simulink model "Hava_Araci_6DOF"  (R2022a)
settings: Solver=ode4  StartTime=0.0  StopTime=inf  FixedStep=1/1000  RelTol=1e-3
InitFcn:
  | addpath(genpath(cd))
  | run('Konfig_Yukle.m')
undefined symbols (not defined in the file or in its folder): aerodatabase, ataletsel, baslangic, e0_0, e1_0, e2_0, e3_0, itki, pm_0, servo, sevo, Vm_0, xme_0
libraries: simulink_extras x9, sharedtransform x3, matrix_library x2, vrlib x1, aerolibtransform2 x1, aerolibatmos2 x1, dspnetwork x1
settings Model: Creator=Fatabi  LastModifiedBy=Fatabi

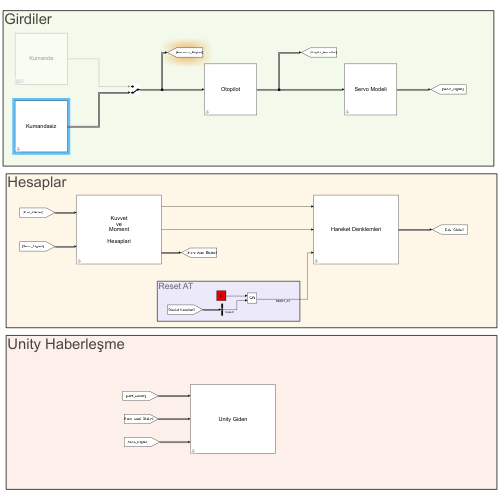
[thumbnail: Simulink's stored preview of the top-level diagram]
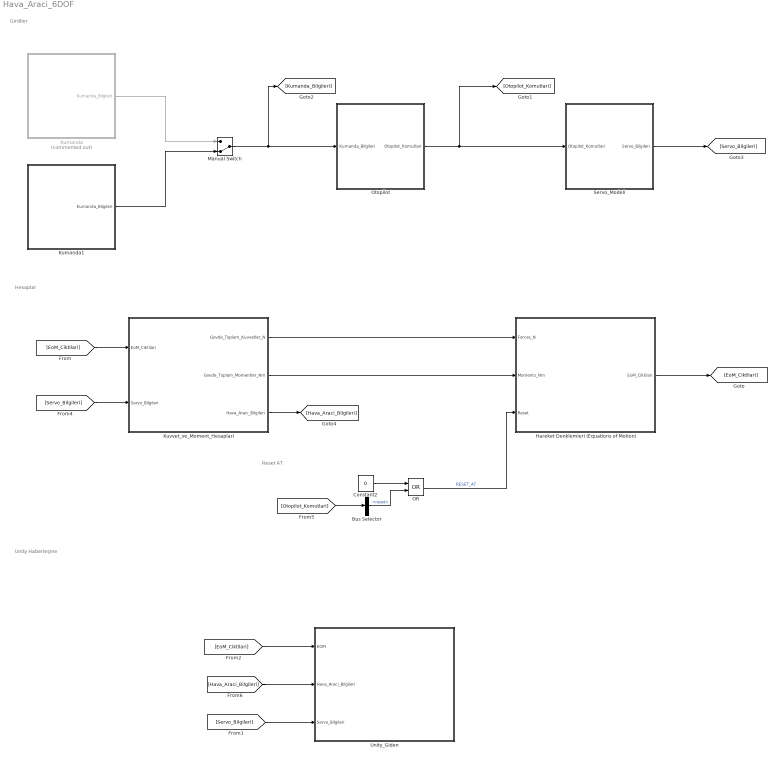
== system Hava_Araci_6DOF ==
  note: Reset AT
  note: Girdiler
  note: Hesaplar
  note: Unity Haberleşme
  Bus Selector : BusSelector  OutputSignals=reset
  Constant2 : Constant  Value=0
      settings: OpenFcn=|
      | val = get_param(gcb,'Value')
      | if val == ('1')
      |    val = '0'
      |    set_param(gcb,'BackgroundColor','red')
      |    set_param(gcb,'Value',val)
      | else
      |    val = '1'
      |    set_param(gcb,'BackgroundColor','green')
      |    set_param(gcb,'Value',val)
      | end
  Hareket Denklemleri (Equations of Motion) : Subsystem
      mask Display: disp('Hareket Denklemleri')
  Kumanda : Subsystem  Commented=on
      mask Display: disp('Kumanda')
  Kumanda1 : Subsystem
      mask Display: disp('Kumandasiz')
  Kuvvet_ve_Moment_Hesaplari : Subsystem
      mask Display: disp(sprintf('Kuvvet\nve\nMoment\n\nHesaplari'))
  Manual Switch : ManualSwitch  CurrentSetting=0
  OR : Logic  Operator=OR  AllPortsSameDT=off  OutDataTypeStr=boolean
  Otopilot : Subsystem
      mask Display: disp('Otopilot');
  Servo_Modeli : Subsystem
      mask Display: disp('Servo Modeli')
  Unity_Giden : Subsystem
      mask Display: disp('Unity Giden')
  wires:
  Hareket Denklemleri (Equations of Motion)/1(EoM_Ciktilari) -> [EoM_Ciktilari]
  Constant2/1 -> OR/1
  [EoM_Ciktilari] -> Unity_Giden/1(EOM)
  [EoM_Ciktilari] -> Kuvvet_ve_Moment_Hesaplari/1(EoM_Ciktilari)
  Kuvvet_ve_Moment_Hesaplari/1(Govde_Toplam_Kuvvetler_N) -> Hareket Denklemleri (Equations of Motion)/1(Forces_N)
  Kuvvet_ve_Moment_Hesaplari/2(Govde_Toplam_Momentler_Nm) -> Hareket Denklemleri (Equations of Motion)/2(Moments_Nm)
  [Servo_Bilgileri] -> Kuvvet_ve_Moment_Hesaplari/2(Servo_Bilgileri)
  Otopilot/1(Otopilot_Komutlari) -> Servo_Modeli/1(Otopilot_Komutlari), [Otopilot_Komutlari]
  Servo_Modeli/1(Servo_Bilgileri) -> [Servo_Bilgileri]
  OR/1 -> Hareket Denklemleri (Equations of Motion)/3(Reset)  "RESET_AT"
  [Otopilot_Komutlari] -> Bus Selector/1
  Bus Selector/1 -> OR/2  "<reset>"
  Kuvvet_ve_Moment_Hesaplari/3(Hava_Araci_Bilgileri) -> [Hava_Araci_Bilgileri]
  [Hava_Araci_Bilgileri] -> Unity_Giden/2(Hava_Araci_Bilgileri)
  [Servo_Bilgileri] -> Unity_Giden/3(Servo_Bilgileri)
  Manual Switch/1 -> [Kumanda_Bilgileri], Otopilot/1(Kumanda_Bilgileri)
  Kumanda/1(Kumanda_Bilgileri) -> Manual Switch/1
  Kumanda1/1(Kumanda_Bilgileri) -> Manual Switch/2

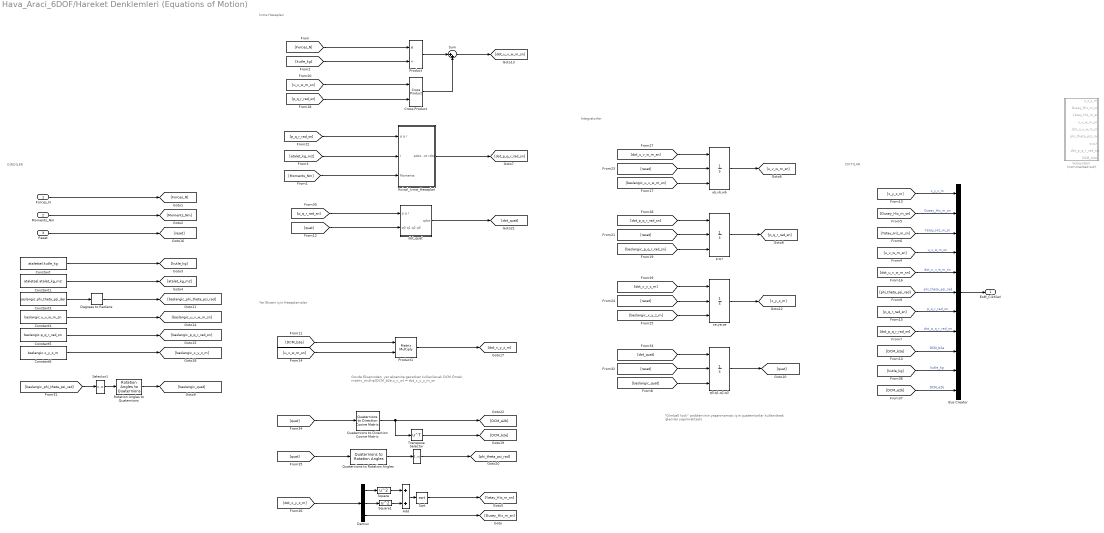
== system Hava_Araci_6DOF/Hareket Denklemleri (Equations of Motion) ==
  note: Govde Ekseninden, yer eksenine gecerken kullanilacak DCM
      |
      | Örnek;
      | matrix_multip(DCM_b2e,u_v_w) = dot_x_y_z_m_sn
  note: İntegratorler
  note: CIKTILAR
  note: GİRDİLER
  note: Yer Ekseni için Hesaplamalar
  note: İvme Hesapları
  note: "Gimball lock" probleminin yaşanmaması için quaternionlar kullanılarak işlemler yapılmaktadır.
  Forces_N : Inport  OutDataTypeStr=double
  Moments_Nm : Inport  Port=2  OutDataTypeStr=double
  Reset : Inport  Port=3
  Acisal_Ivme_Hesaplari : Subsystem
  Add : Sum
  Bus Creator : BusCreator  Inputs=11
  Constant : Constant  Value=ataletsel.kutle_kg  OutDataTypeStr=Inherit: Inherit via back propagation
  Constant1 : Constant  Value=ataletsel.atalet_kg_m2  OutDataTypeStr=Inherit: Inherit via back propagation
  Constant3 : Constant  Value=baslangic.phi_theta_psi_der  OutDataTypeStr=Inherit: Inherit via back propagation
  Constant4 : Constant  Value=baslangic.u_v_w_m_sn  OutDataTypeStr=Inherit: Inherit via back propagation
  Constant5 : Constant  Value=baslangic.p_q_r_rad_sn  OutDataTypeStr=Inherit: Inherit via back propagation
  Constant6 : Constant  Value=baslangic.x_y_z_m  OutDataTypeStr=Inherit: Inherit via back propagation
  Cross Product : matrix_library/Cross Product
      settings: SourceProductBaseCode=SL
  Degrees to Radians : simulink_extras/Transformations/Degrees to Radians
  Demux : Demux  Outputs=3
  Product : Product  Inputs=*/  SaturateOnIntegerOverflow=on  OutDataTypeStr=Inherit: Same as first input
  Product1 : Product  Multiplication=Matrix(*)
  Quaternions to Direction Cosine Matrix : sharedtransform/Quaternions to  Direction Cosine Matrix  aMode=aMode
      settings: SourceProductBaseCode=AE,PW,DR,MT,VE
  Quaternions to Rotation Angles : sharedtransform/Quaternions to Rotation Angles  rotationOrder=ZYX  aMode=aMode
      settings: SourceProductBaseCode=AE,PW,DR,MT,VE
  Rotation Angles to Quaternions : sharedtransform/Rotation Angles to Quaternions  rotationOrder=ZYX  aMode=aMode
      settings: SourceProductBaseCode=AE,PW,DR,MT,VE
  Selector : Selector  InputPortWidth=3  IndexOptions=Index vector (dialog)  Indices=[3 2 1]  OutputSizes=1
  Selector1 : Selector  InputPortWidth=3  IndexOptions=Index vector (dialog)  Indices=[3 2 1]  OutputSizes=1
  Sqrt : Sqrt
  Square : Math  Operator=square
  Square1 : Math  Operator=square
  Subsystem : Subsystem  Commented=on
  Sum : Sum  Inputs=|++  SaturateOnIntegerOverflow=on
  Transpose : Math  Operator=transpose  SignedPower=on
  dot_quat : Subsystem
  "p,q,r " : Integrator  ExternalReset=rising  InitialConditionSource=external  InitialCondition=pm_0
  q0,q1,q2,q3 : Integrator  ExternalReset=rising  InitialConditionSource=external  InitialCondition=[e0_0 e1_0 e2_0 e3_0]
  ub,vb,wb : Integrator  ExternalReset=rising  InitialConditionSource=external  InitialCondition=Vm_0
  xe,ye,ze : Integrator  ExternalReset=rising  InitialConditionSource=external  InitialCondition=xme_0
  EoM_Ciktilari : Outport
  wires:
  ub,vb,wb/1 -> [u_v_w_m_sn]
  Sum/1 -> [dot_u_v_w_m_sn]
  "p,q,r "/1 -> [p_q_r_rad_sn]
  [Forces_N] -> Product/1
  Acisal_Ivme_Hesaplari/1(pdot qdot rdot) -> [dot_p_q_r_rad_sn]
  [kutle_kg] -> Product/2
  Product/1 -> Sum/1
  [Moments_Nm] -> Acisal_Ivme_Hesaplari/3(Moments)
  Cross Product/1 -> Sum/2
  Product1/1 -> [dot_x_y_z_m]
  [atalet_kg_m2] -> Acisal_Ivme_Hesaplari/2(I)
  Forces_N/1 -> [Forces_N]
  Moments_Nm/1 -> [Moments_Nm]
  Constant/1 -> [kutle_kg]
  Constant1/1 -> [atalet_kg_m2]
  Demux/1 -> Square/1
  Demux/2 -> Square1/1
  Demux/3 -> [Dusey_Hiz_m_sn]
  Square/1 -> Add/1
  Square1/1 -> Add/2
  Add/1 -> Sqrt/1
  Sqrt/1 -> [Yatay_Hiz_m_sn]
  Constant3/1 -> Degrees to Radians/1
  Degrees to Radians/1 -> [baslangic_phi_theta_psi_rad]
  xe,ye,ze/1 -> [x_y_z_m]
  [baslangic_u_v_w_m_sn] -> ub,vb,wb/3
  Constant4/1 -> [baslangic_u_v_w_m_sn]
  [p_q_r_rad_sn] -> Cross Product/2
  Constant5/1 -> [baslangic_p_q_r_rad_sn]
  [baslangic_p_q_r_rad_sn] -> "p,q,r "/3
  [u_v_w_m_sn] -> Cross Product/1
  Reset/1 -> [reset]
  [p_q_r_rad_sn] -> Acisal_Ivme_Hesaplari/1(p q r)
  Constant6/1 -> [baslangic_x_y_z_m]
  [baslangic_x_y_z_m] -> xe,ye,ze/3
  [dot_x_y_z_m] -> Demux/1
  [dot_u_v_w_m_sn] -> ub,vb,wb/1
  [dot_p_q_r_rad_sn] -> "p,q,r "/1
  [dot_x_y_z_m] -> xe,ye,ze/1
  [DCM_b2e] -> Product1/1
  Transpose/1 -> [DCM_b2e]
  Quaternions to Rotation Angles/1 -> Selector/1
  Quaternions to Direction Cosine Matrix/1 -> [DCM_e2b], Transpose/1
  q0,q1,q2,q3/1 -> [quat]
  Selector/1 -> [phi_theta_psi_rad]
  [dot_quat] -> q0,q1,q2,q3/1
  [baslangic_phi_theta_psi_rad] -> Selector1/1
  Selector1/1 -> Rotation Angles to Quaternions/1
  Rotation Angles to Quaternions/1 -> [baslangic_quat]
  [baslangic_quat] -> q0,q1,q2,q3/3
  [quat] -> dot_quat/2(q0 q1 q2 q3)
  [p_q_r_rad_sn] -> dot_quat/1(p q r)
  dot_quat/1(qdot) -> [dot_quat]
  [quat] -> Quaternions to Direction Cosine Matrix/1
  [quat] -> Quaternions to Rotation Angles/1
  [reset] -> ub,vb,wb/2
  [reset] -> "p,q,r "/2
  [reset] -> xe,ye,ze/2
  [reset] -> q0,q1,q2,q3/2
  [x_y_z_m] -> Bus Creator/1  "x_y_z_m"
  [Dusey_Hiz_m_sn] -> Bus Creator/2  "Dusey_Hiz_m_sn"
  [Yatay_Hiz_m_sn] -> Bus Creator/3  "Yatay_Hiz_m_sn"
  [u_v_w_m_sn] -> Bus Creator/4  "u_v_w_m_sn"
  [dot_u_v_w_m_sn] -> Bus Creator/5  "dot_u_v_w_m_sn"
  [phi_theta_psi_rad] -> Bus Creator/6  "phi_theta_psi_rad"
  [p_q_r_rad_sn] -> Bus Creator/7  "p_q_r_rad_sn"
  [dot_p_q_r_rad_sn] -> Bus Creator/8  "dot_p_q_r_rad_sn"
  [DCM_b2e] -> Bus Creator/9  "DCM_b2e"
  Bus Creator/1 -> EoM_Ciktilari/1
  [u_v_w_m_sn] -> Product1/2
  [kutle_kg] -> Bus Creator/10  "kutle_kg"
  [DCM_e2b] -> Bus Creator/11  "DCM_e2b"

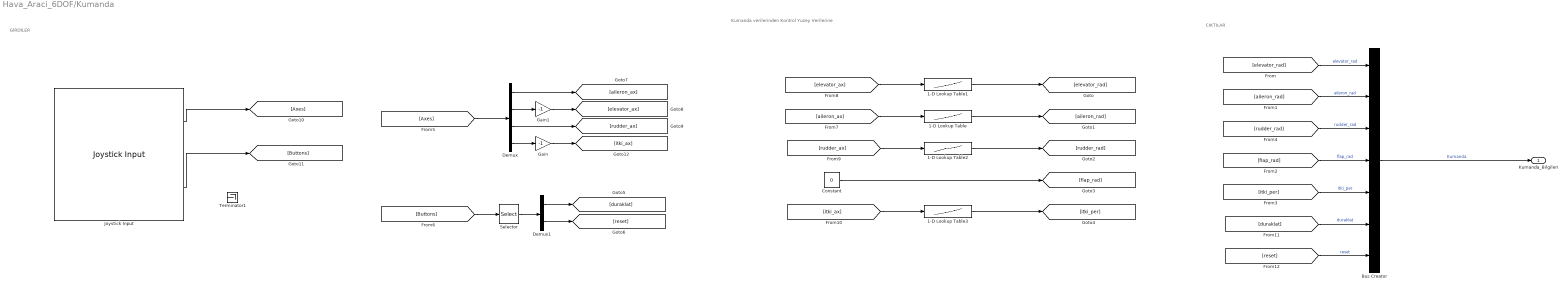
== system Hava_Araci_6DOF/Kumanda ==
  note: CIKTILAR
  note: GİRDİLER
  note: Kumanda verilerinden Kontrol Yuzey Verilerine
  1-D Lookup Table : Lookup_n-D  NumberOfTableDimensions=1  BreakpointsForDimension1=[-1,1]  Table=servo.aileron.limitler.aci_rad  ExtrapMethod=Clip  InternalRulePriority=Speed  RndMeth=Simplest
  1-D Lookup Table1 : Lookup_n-D  NumberOfTableDimensions=1  BreakpointsForDimension1=[-1,1]  Table=servo.elevator.limitler.aci_rad  ExtrapMethod=Clip  InternalRulePriority=Speed  RndMeth=Simplest
  1-D Lookup Table2 : Lookup_n-D  NumberOfTableDimensions=1  BreakpointsForDimension1=[-1,1]  Table=servo.rudder.limitler.aci_rad  ExtrapMethod=Clip  InternalRulePriority=Speed  RndMeth=Simplest
  1-D Lookup Table3 : Lookup_n-D  NumberOfTableDimensions=1  BreakpointsForDimension1=[-1,1]  Table=servo.thrust.limitler.itki_yuzde_per  ExtrapMethod=Clip  InternalRulePriority=Speed  RndMeth=Simplest
  Bus Creator : BusCreator  Inputs=7
  Constant : Constant  Value=0
  Demux : Demux
  Demux1 : Demux  Outputs=2
  Gain : Gain  Gain=-1
  Gain1 : Gain  Gain=-1
  Joystick Input : vrlib/Joystick Input  joyid=1  adjustports=on  forcefeed=off
  Selector : Selector  IndexOptions=Index vector (dialog)  Indices=[1,2]  OutputSizes=1
  Terminator1 : Terminator
  Kumanda_Bilgileri : Outport
  wires:
  [aileron_rad] -> Bus Creator/2  "aileron_rad"
  [elevator_rad] -> Bus Creator/1  "elevator_rad"
  [rudder_rad] -> Bus Creator/3  "rudder_rad"
  [flap_rad] -> Bus Creator/4  "flap_rad"
  [itki_per] -> Bus Creator/5  "itki_per"
  Bus Creator/1 -> Kumanda_Bilgileri/1  "Kumanda"
  Joystick Input/1 -> [Axes]
  ? -> Terminator1/1
  Joystick Input/2 -> [Buttons]
  Selector/1 -> Demux1/1
  Demux1/1 -> [duraklat]
  Demux1/2 -> [reset]
  Demux/1 -> [aileron_ax]
  Demux/2 -> Gain1/1
  Demux/3 -> [rudder_ax]
  [Axes] -> Demux/1
  [Buttons] -> Selector/1
  Demux/4 -> Gain/1
  Gain/1 -> [itki_ax]
  Constant/1 -> [flap_rad]
  [elevator_ax] -> 1-D Lookup Table1/1
  [aileron_ax] -> 1-D Lookup Table/1
  [rudder_ax] -> 1-D Lookup Table2/1
  [itki_ax] -> 1-D Lookup Table3/1
  1-D Lookup Table1/1 -> [elevator_rad]
  1-D Lookup Table/1 -> [aileron_rad]
  1-D Lookup Table2/1 -> [rudder_rad]
  1-D Lookup Table3/1 -> [itki_per]
  [duraklat] -> Bus Creator/6  "duraklat"
  [reset] -> Bus Creator/7  "reset"
  Gain1/1 -> [elevator_ax]

== system Hava_Araci_6DOF/Kumanda1 ==
  note: Kumanda verilerinden Kontrol Yuzey Verilerine
  note: CIKTILAR
  Bus Creator : BusCreator  Inputs=7
  Constant : Constant  Value=[0,0,0,0,50,0,0]
  Demux : Demux  Outputs=7
  Kumanda_Bilgileri : Outport
  wires:
  [reset] -> Bus Creator/7  "reset"
  [duraklat] -> Bus Creator/6  "duraklat"
  Bus Creator/1 -> Kumanda_Bilgileri/1  "Kumanda"
  [itki_per] -> Bus Creator/5  "itki_per"
  [flap_rad] -> Bus Creator/4  "flap_rad"
  [rudder_rad] -> Bus Creator/3  "rudder_rad"
  [elevator_rad] -> Bus Creator/1  "elevator_rad"
  [aileron_rad] -> Bus Creator/2  "aileron_rad"
  Constant/1 -> Demux/1
  Demux/1 -> [elevator_rad]
  Demux/2 -> [aileron_rad]
  Demux/3 -> [rudder_rad]
  Demux/4 -> [flap_rad]
  Demux/5 -> [itki_per]
  Demux/6 -> [duraklat]
  Demux/7 -> [reset]

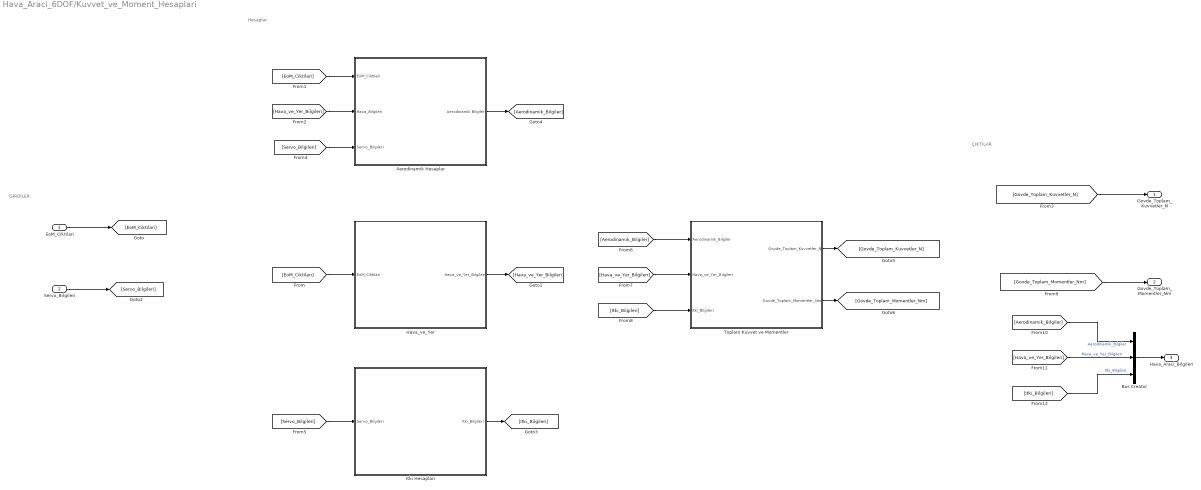
== system Hava_Araci_6DOF/Kuvvet_ve_Moment_Hesaplari ==
  note: GİRDİLER
  note: ÇIKTILAR
  note: Hesaplar
  EoM_Ciktilari : Inport
  Servo_Bilgileri : Inport  Port=2
  Aerodinamik Hesaplar : Subsystem
  Bus Creator : BusCreator  Inputs=3
  Hava_ve_Yer : Subsystem
  Itki Hesapları : Subsystem
  Toplam Kuvvet ve Momentler : Subsystem
  Govde_Toplam_Kuvvetler_N : Outport
  Govde_Toplam_Momentler_Nm : Outport  Port=2
  Hava_Araci_Bilgileri : Outport  Port=3
  wires:
  [Hava_ve_Yer_Bilgileri] -> Aerodinamik Hesaplar/2(Hava_Bilgileri)
  EoM_Ciktilari/1 -> [EoM_Ciktilari]
  [EoM_Ciktilari] -> Hava_ve_Yer/1(EoM_Ciktilari)
  [EoM_Ciktilari] -> Aerodinamik Hesaplar/1(EoM_Ciktilari)
  Hava_ve_Yer/1(Hava_ve_Yer_Bilgileri) -> [Hava_ve_Yer_Bilgileri]
  Servo_Bilgileri/1 -> [Servo_Bilgileri]
  [Servo_Bilgileri] -> Aerodinamik Hesaplar/3(Servo_Bilgileri)
  [Servo_Bilgileri] -> Itki Hesapları/1(Servo_Bilgileri)
  Itki Hesapları/1(Itki_Bilgileri) -> [Itki_Bilgileri]
  Aerodinamik Hesaplar/1(Aerodinamik Bilgiler) -> [Aerodinamik_Bilgiler]
  [Aerodinamik_Bilgiler] -> Toplam Kuvvet ve Momentler/1(Aerodinamik_Bilgiler)
  [Hava_ve_Yer_Bilgileri] -> Toplam Kuvvet ve Momentler/2(Hava_ve_Yer_Bilgileri)
  [Itki_Bilgileri] -> Toplam Kuvvet ve Momentler/3(Itki_Bilgileri)
  Toplam Kuvvet ve Momentler/1(Govde_Toplam_Kuvvetler_N) -> [Govde_Toplam_Kuvvetler_N]
  Toplam Kuvvet ve Momentler/2(Govde_Toplam_Momentler_Nm) -> [Govde_Toplam_Momentler_Nm]
  [Govde_Toplam_Momentler_Nm] -> Govde_Toplam_Momentler_Nm/1
  [Govde_Toplam_Kuvvetler_N] -> Govde_Toplam_Kuvvetler_N/1
  [Hava_ve_Yer_Bilgileri] -> Bus Creator/2  "Hava_ve_Yer_Bilgileri"
  [Aerodinamik_Bilgiler] -> Bus Creator/1  "Aerodinamik_Bilgiler"
  [Itki_Bilgileri] -> Bus Creator/3  "Itki_Bilgileri"
  Bus Creator/1 -> Hava_Araci_Bilgileri/1

== system Hava_Araci_6DOF/Otopilot ==
  note: SUAN SADECE KUMANDA ile CALISMAKTADIR.
  Kumanda_Bilgileri : Inport
  Bus Creator : BusCreator  Inputs=7
  Bus Selector : BusSelector  OutputSignals=elevator_rad,aileron_rad,rudder_rad,flap_rad,itki_per,duraklat,reset
  Otopilot_Komutlari : Outport
  wires:
  Bus Creator/1 -> Otopilot_Komutlari/1  "Otopilot_Servo_Komutlari"
  [itki_per] -> Bus Creator/5  "itki_per"
  [flap_rad] -> Bus Creator/4  "flap_rad"
  [rudder_rad] -> Bus Creator/3  "rudder_rad"
  [elevator_rad] -> Bus Creator/1  "elevator_rad"
  [aileron_rad] -> Bus Creator/2  "aileron_rad"
  Kumanda_Bilgileri/1 -> Bus Selector/1
  Bus Selector/2 -> [aileron_rad]  "<aileron_rad>"
  Bus Selector/1 -> [elevator_rad]  "<elevator_rad>"
  Bus Selector/3 -> [rudder_rad]  "<rudder_rad>"
  Bus Selector/4 -> [flap_rad]  "<flap_rad>"
  Bus Selector/5 -> [itki_per]  "<itki_per>"
  Bus Selector/6 -> [duraklat]  "<duraklat>"
  Bus Selector/7 -> [reset]  "<reset>"
  [duraklat] -> Bus Creator/6  "duraklat"
  [reset] -> Bus Creator/7  "reset"

== system Hava_Araci_6DOF/Servo_Modeli ==
  Otopilot_Komutlari : Inport
  Bus Creator : BusCreator  Inputs=5
  Bus Selector : BusSelector  OutputSignals=elevator_rad,aileron_rad,rudder_rad,flap_rad,itki_per
  Rate Limiter : RateLimiter  RisingSlewLimit=servo.aileron.limitler.acisal_hiz_rad_sn(2)  FallingSlewLimit=servo.aileron.limitler.acisal_hiz_rad_sn(1)  SampleTimeMode=inherited
  Rate Limiter1 : RateLimiter  RisingSlewLimit=servo.elevator.limitler.acisal_hiz_rad_sn(2)  FallingSlewLimit=servo.elevator.limitler.acisal_hiz_rad_sn(1)  SampleTimeMode=inherited
  Rate Limiter2 : RateLimiter  RisingSlewLimit=servo.rudder.limitler.acisal_hiz_rad_sn(2)  FallingSlewLimit=servo.rudder.limitler.acisal_hiz_rad_sn(1)  SampleTimeMode=inherited
  Rate Limiter3 : RateLimiter  RisingSlewLimit=servo.thrust.limitler.itki_hizi_per_sn(2)  FallingSlewLimit=servo.thrust.limitler.itki_hizi_per_sn(1)  SampleTimeMode=inherited
  Rate Limiter4 : RateLimiter  RisingSlewLimit=sevo.flap.limitler.acisal_hiz_rad_sn(2)  FallingSlewLimit=sevo.flap.limitler.acisal_hiz_rad_sn(1)  SampleTimeMode=inherited
  Servo_Bilgileri : Outport
  wires:
  [aileron_rad] -> Bus Creator/2  "aileron_rad"
  [elevator_rad] -> Bus Creator/1  "elevator_rad"
  [rudder_rad] -> Bus Creator/3  "rudder_rad"
  [flap_rad] -> Bus Creator/4  "flap_rad"
  [itki_per] -> Bus Creator/5  "itki_per"
  Bus Creator/1 -> Servo_Bilgileri/1  "Servo"
  Rate Limiter/1 -> [elevator_rad]
  Rate Limiter1/1 -> [aileron_rad]
  Rate Limiter2/1 -> [rudder_rad]
  Rate Limiter3/1 -> [itki_per]
  Otopilot_Komutlari/1 -> Bus Selector/1
  Bus Selector/1 -> Rate Limiter/1  "<elevator_rad>"
  Bus Selector/2 -> Rate Limiter1/1  "<aileron_rad>"
  Bus Selector/3 -> Rate Limiter2/1  "<rudder_rad>"
  Bus Selector/5 -> Rate Limiter3/1  "<itki_per>"
  Bus Selector/4 -> Rate Limiter4/1  "<flap_rad>"
  Rate Limiter4/1 -> [flap_rad]

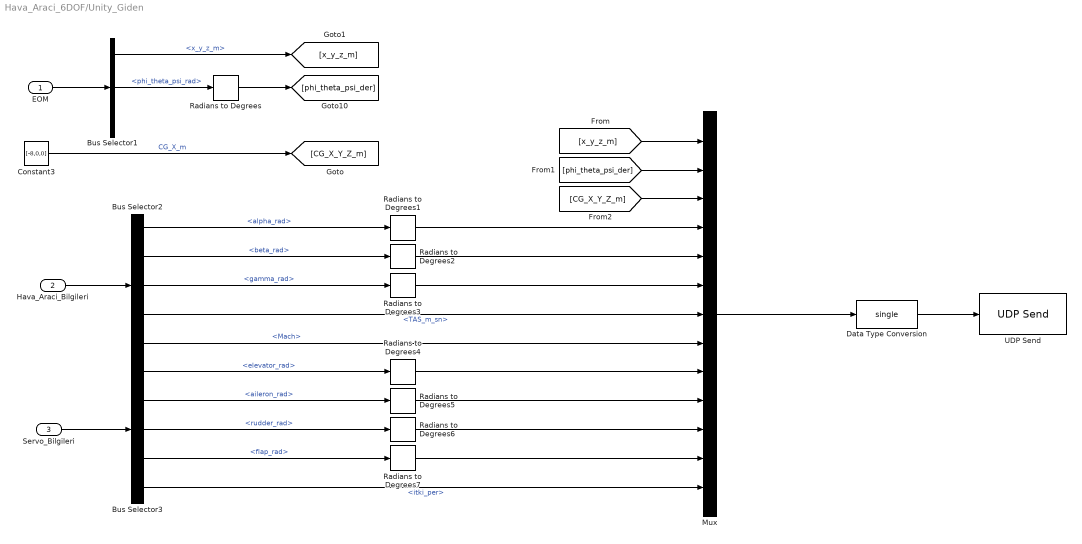
== system Hava_Araci_6DOF/Unity_Giden ==
  EOM : Inport
  Hava_Araci_Bilgileri : Inport  Port=2
  Servo_Bilgileri : Inport  Port=3
  Bus Selector1 : BusSelector  OutputSignals=x_y_z_m,phi_theta_psi_rad,Dusey_Hiz_m_sn
  Bus Selector2 : BusSelector  OutputSignals=Hava_ve_Yer_Bilgileri.alpha_rad,Hava_ve_Yer_Bilgileri.beta_rad,Hava_ve_Yer_Bilgileri.gamma_rad,Hava_ve_Yer_Bilgileri.TAS_m_sn,Hava_ve_Yer_Bilgileri.Mach
  Bus Selector3 : BusSelector  OutputSignals=elevator_rad,aileron_rad,rudder_rad,flap_rad,itki_per
  Constant3 : Constant  Value=[-8,0,0]
  Data Type Conversion : DataTypeConversion  OutDataTypeStr=single  SaturateOnIntegerOverflow=off  RndMeth=Floor
  Mux : Mux  Inputs=13
  Radians to Degrees{,1..7} (8 alike) : simulink_extras/Transformations/Radians to Degrees
  UDP Send : dspnetwork/UDP Send  remoteURL='127.0.0.1'  remotePort=8001  localURL='0.0.0.0'  localPortSource=Automatically determine  localPort=-1  sendBufferSize=76  sampletime=-1  blockPlatform=[]  separateLengthPort=0
  wires:
  Mux/1 -> Data Type Conversion/1
  Data Type Conversion/1 -> UDP Send/1
  Bus Selector1/1 -> [x_y_z_m]  "<x_y_z_m>"
  EOM/1 -> Bus Selector1/1
  Constant3/1 -> [CG_X_Y_Z_m]  "CG_X_m"
  [x_y_z_m] -> Mux/1
  Bus Selector1/2 -> Radians to Degrees/1  "<phi_theta_psi_rad>"
  Radians to Degrees/1 -> [phi_theta_psi_der]
  [phi_theta_psi_der] -> Mux/2
  [CG_X_Y_Z_m] -> Mux/3
  Hava_Araci_Bilgileri/1 -> Bus Selector2/1
  Servo_Bilgileri/1 -> Bus Selector3/1
  Bus Selector2/5 -> Mux/8  "<Mach>"
  Bus Selector2/4 -> Mux/7  "<TAS_m_sn>"
  Bus Selector2/3 -> Radians to Degrees3/1  "<gamma_rad>"
  Bus Selector2/2 -> Radians to Degrees2/1  "<beta_rad>"
  Bus Selector2/1 -> Radians to Degrees1/1  "<alpha_rad>"
  Bus Selector3/1 -> Radians to Degrees4/1  "<elevator_rad>"
  Bus Selector3/2 -> Radians to Degrees5/1  "<aileron_rad>"
  Bus Selector3/3 -> Radians to Degrees6/1  "<rudder_rad>"
  Bus Selector3/4 -> Radians to Degrees7/1  "<flap_rad>"
  Bus Selector3/5 -> Mux/13  "<itki_per>"
  Radians to Degrees1/1 -> Mux/4
  Radians to Degrees2/1 -> Mux/5
  Radians to Degrees3/1 -> Mux/6
  Radians to Degrees4/1 -> Mux/9
  Radians to Degrees5/1 -> Mux/10
  Radians to Degrees6/1 -> Mux/11
  Radians to Degrees7/1 -> Mux/12

== system Hava_Araci_6DOF/Hareket Denklemleri (Equations of Motion)/Acisal_Ivme_Hesaplari ==
  note: GİRDİLER
  note: ÇIKTILAR
  note: Açısal İvme Hesapları
  p q r : Inport  OutDataTypeStr=double
  I : Inport  Port=2  OutDataTypeStr=double
  Moments : Inport  Port=3  OutDataTypeStr=double
  Add : Sum  Inputs=+-
  Cross Product : matrix_library/Cross Product
      settings: SourceProductBaseCode=SL
  Product2 : Product  Inputs=*/  Multiplication=Matrix(*)  SaturateOnIntegerOverflow=on  OutDataTypeStr=Inherit: Same as first input
  Reshape : Reshape
  Reshape1 : Reshape  OutputDimensionality=Row vector (2-D)
  Subsystem : Subsystem
  pdot qdot rdot : Outport  OutDataTypeStr=double  VectorParamsAs1DForOutWhenUnconnected=off
  wires:
  Add/1 -> Reshape1/1
  Subsystem/1(I * w) -> Cross Product/2
  [p_q_r_rad_sn] -> Subsystem/1(p q r), Cross Product/1
  Cross Product/1 -> Add/2
  Product2/1 -> Reshape/1
  Reshape/1 -> pdot qdot rdot/1
  Reshape1/1 -> Product2/1
  [I] -> Subsystem/2(Inertia)
  [Moments] -> Add/1
  [I] -> Product2/2
  p q r/1 -> [p_q_r_rad_sn]
  Moments/1 -> [Moments]
  I/1 -> [I]

== system Hava_Araci_6DOF/Hareket Denklemleri (Equations of Motion)/Subsystem ==
  x_y_z_m : Outport  OutDataTypeStr=double  Unit=m  VectorParamsAs1DForOutWhenUnconnected=off
  Dusey_Hiz_m_sn : Outport  Port=2  OutDataTypeStr=double  Unit=m/s  VectorParamsAs1DForOutWhenUnconnected=off
  Yatay_Hiz_m_sn : Outport  Port=3  OutDataTypeStr=double  Unit=m/s  VectorParamsAs1DForOutWhenUnconnected=off
  u_v_w_m_sn : Outport  Port=4  OutDataTypeStr=double  Unit=m/s  VectorParamsAs1DForOutWhenUnconnected=off
  dot_u_v_w_m_sn : Outport  Port=5  OutDataTypeStr=double  Unit=m/s^2  VectorParamsAs1DForOutWhenUnconnected=off
  phi_theta_psi_rad : Outport  Port=6  OutDataTypeStr=double  Unit=rad  VectorParamsAs1DForOutWhenUnconnected=off
  p,q,r : Outport  Port=7  OutDataTypeStr=double  Unit=rad/s  VectorParamsAs1DForOutWhenUnconnected=off
  dot_p_q_r_rad_sn : Outport  Port=8  OutDataTypeStr=double  Unit=rad/s^2  VectorParamsAs1DForOutWhenUnconnected=off
  DCM_b2e : Outport  Port=9  OutDataTypeStr=double  Unit=1  VectorParamsAs1DForOutWhenUnconnected=off

== system Hava_Araci_6DOF/Hareket Denklemleri (Equations of Motion)/dot_quat ==
  p q r : Inport
  q0 q1 q2 q3 : Inport  Port=2
  Constant : Constant
  Dot Product : DotProduct  InputSameDT=off  OutDataTypeStr=Inherit: Inherit via internal rule
  High Gain Quaternion Normalization : Gain  SaturateOnIntegerOverflow=on  OutDataTypeStr=Inherit: Same as input  ParamDataTypeStr=Inherit: Same as input
  Mux1 : Mux  Inputs=[3 4 1]
  Mux2 : Mux
  Sum : Sum  Inputs=|+-  InputSameDT=on  SaturateOnIntegerOverflow=on  OutDataTypeStr=Inherit: Same as first input
  q0dot : Fcn  Expr=-0.5 * ( u[5]*u[1]+u[6]*u[2]+u[7]*u[3] ) + u[8]*u[4]
  q1dot : Fcn  Expr=0.5 * ( u[4]*u[1]+u[6]*u[3]-u[7]*u[2] ) + u[8]*u[5]
  q2dot : Fcn  Expr=0.5 * ( u[4]*u[2]+u[7]*u[1]-u[5]*u[3] ) + u[8]*u[6]
  q3dot : Fcn  Expr=0.5 * ( u[4]*u[3]+u[5]*u[2]-u[6]*u[1] ) + u[8]*u[7]
  qdot : Outport  InitialOutput=0  VectorParamsAs1DForOutWhenUnconnected=off
  wires:
  Dot Product/1 -> Sum/2
  p q r/1 -> Mux1/1
  Mux1/1 -> q2dot/1, q3dot/1, q0dot/1, q1dot/1
  High Gain Quaternion Normalization/1 -> Mux1/3
  q2dot/1 -> Mux2/3
  Constant/1 -> Sum/1
  q1dot/1 -> Mux2/2
  Mux2/1 -> qdot/1
  Sum/1 -> High Gain Quaternion Normalization/1
  q0 q1 q2 q3/1 -> Dot Product/1, Dot Product/2, Mux1/2
  q3dot/1 -> Mux2/4
  q0dot/1 -> Mux2/1

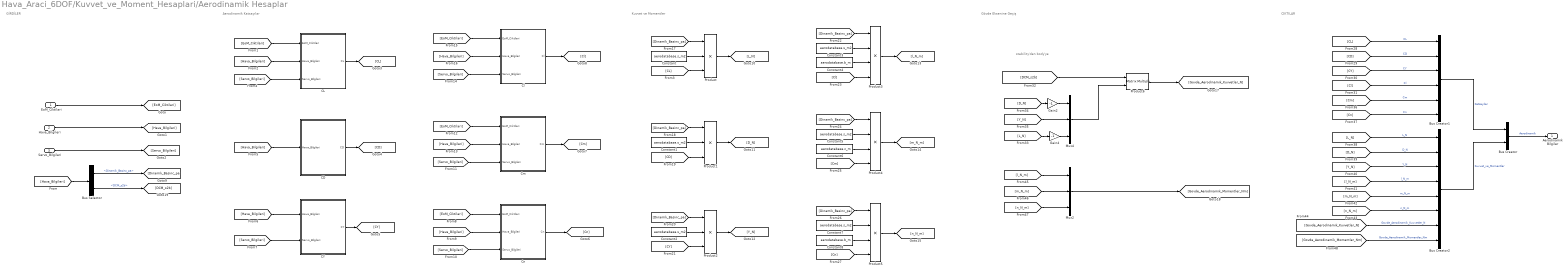
== system Hava_Araci_6DOF/Kuvvet_ve_Moment_Hesaplari/Aerodinamik Hesaplar ==
  note: Aerodinamik Katsayılar
  note: CIKTILAR
  note: GİRDİLER
  note: Kuvvet ve Momentler
  note: Gövde Eksenine Geçiş
  note: stability'den body'ye
  EoM_Ciktilari : Inport  OutDataTypeStr=double
  Hava_Bilgileri : Inport  Port=2
  Servo_Bilgileri : Inport  Port=3
  Bus Creator : BusCreator  Inputs=2
  Bus Creator1 : BusCreator  Inputs=6
  Bus Creator2 : BusCreator  Inputs=8
  Bus Selector : BusSelector  OutputSignals=Dinamik_Basinc_pa,DCM_s2b
  CD : Subsystem
  CL : Subsystem
  CY : Subsystem
  Cl : Subsystem
  Cm : Subsystem
  Cn : Subsystem
  Constant{,1..3,5,7} (6 alike) : Constant  Value=aerodatabase.s_m2
  Constant4 : Constant  Value=aerodatabase.b_m
  Constant6 : Constant  Value=aerodatabase.c_m
  Constant8 : Constant  Value=aerodatabase.b_m
  Gain2 : Gain  Gain=-1
  Gain4 : Gain  Gain=-1
  Mux2 : Mux  Inputs=3
  Mux4 : Mux  Inputs=3
  Product : Product  Inputs=3
  Product1 : Product  Inputs=3
  Product2 : Product  Inputs=3
  Product3 : Product  Inputs=4
  Product4 : Product  Inputs=4
  Product5 : Product  Inputs=4
  Product6 : Product  Multiplication=Matrix(*)
  Aerodinamik Bilgiler : Outport
  wires:
  EoM_Ciktilari/1 -> [EoM_Ciktilari]
  Hava_Bilgileri/1 -> [Hava_Bilgileri]
  Servo_Bilgileri/1 -> [Servo_Bilgileri]
  [EoM_Ciktilari] -> CL/1(EoM_Ciktilari)
  [Hava_Bilgileri] -> CL/2(Hava_Bilgileri)
  [Servo_Bilgileri] -> CL/3(Servo_Bilgileri)
  [Hava_Bilgileri] -> CD/1(Hava_Bilgileri)
  [Servo_Bilgileri] -> CY/2(Servo_Bilgileri)
  [Hava_Bilgileri] -> CY/1(Hava_Bilgileri)
  [EoM_Ciktilari] -> Cn/1(EoM_Ciktilari)
  [Hava_Bilgileri] -> Cn/2(Hava_Bilgileri)
  [Servo_Bilgileri] -> Cn/3(Servo_Bilgileri)
  [EoM_Ciktilari] -> Cm/1(EoM_Ciktilari)
  [Hava_Bilgileri] -> Cm/2(Hava_Bilgileri)
  [Servo_Bilgileri] -> Cm/3(Servo_Bilgileri)
  [Servo_Bilgileri] -> Cl/3(Servo_Bilgileri)
  [Hava_Bilgileri] -> Cl/2(Hava_Bilgileri)
  [EoM_Ciktilari] -> Cl/1(EoM_Ciktilari)
  CL/1(CL) -> [CL]
  CD/1(CD) -> [CD]
  CY/1(CY) -> [CY]
  Cn/1(Cn) -> [Cn]
  Cm/1(Cm) -> [Cm]
  Cl/1(Cl) -> [Cl]
  [Hava_Bilgileri] -> Bus Selector/1
  Bus Selector/1 -> [Dinamik_Basinc_pa]  "<Dinamik_Basinc_pa>"
  [Dinamik_Basinc_pa] -> Product/1
  Constant/1 -> Product/2
  [CL] -> Product/3
  Product/1 -> [L_N]
  Product1/1 -> [D_N]
  [CD] -> Product1/3
  Constant1/1 -> Product1/2
  [Dinamik_Basinc_pa] -> Product1/1
  [Dinamik_Basinc_pa] -> Product2/1
  Constant2/1 -> Product2/2
  [CY] -> Product2/3
  Product2/1 -> [Y_N]
  Product3/1 -> [l_N_m]
  Constant4/1 -> Product3/3
  Constant3/1 -> Product3/2
  [Dinamik_Basinc_pa] -> Product3/1
  [Cl] -> Product3/4
  [Cm] -> Product4/4
  [Dinamik_Basinc_pa] -> Product4/1
  Constant5/1 -> Product4/2
  Constant6/1 -> Product4/3
  Product4/1 -> [m_N_m]
  Product5/1 -> [n_N_m]
  Constant8/1 -> Product5/3
  Constant7/1 -> Product5/2
  [Dinamik_Basinc_pa] -> Product5/1
  [Cn] -> Product5/4
  Bus Selector/2 -> [DCM_s2b]  "<DCM_s2b>"
  [CL] -> Bus Creator1/1  "CL"
  [CD] -> Bus Creator1/2  "CD"
  [CY] -> Bus Creator1/3  "CY"
  [Cl] -> Bus Creator1/4  "Cl"
  [Cm] -> Bus Creator1/5  "Cm"
  [Cn] -> Bus Creator1/6  "Cn"
  Bus Creator1/1 -> Bus Creator/1  "Katsayilar"
  Bus Creator2/1 -> Bus Creator/2  "Kuvvet_ve_Momentler"
  [m_N_m] -> Bus Creator2/5  "m_N_m"
  [l_N_m] -> Bus Creator2/4  "l_N_m"
  [Y_N] -> Bus Creator2/3  "Y_N"
  [D_N] -> Bus Creator2/2  "D_N"
  [L_N] -> Bus Creator2/1  "L_N"
  [n_N_m] -> Bus Creator2/6  "n_N_m"
  [Govde_Aerodinamik_Kuvvetler_N] -> Bus Creator2/7  "Govde_Aerodinamik_Kuvvetler_N"
  Mux2/1 -> [Govde_Aerodinamik_Momentler_Nm]
  [l_N_m] -> Mux2/1
  [m_N_m] -> Mux2/2
  [n_N_m] -> Mux2/3
  [Govde_Aerodinamik_Momentler_Nm] -> Bus Creator2/8  "Govde_Aerodinamik_Momentler_Nm"
  Bus Creator/1 -> Aerodinamik Bilgiler/1  "Aerodinamik"
  [Y_N] -> Mux4/2
  Gain4/1 -> Mux4/3
  [D_N] -> Gain2/1
  Mux4/1 -> Product6/2
  Gain2/1 -> Mux4/1
  [L_N] -> Gain4/1
  Product6/1 -> [Govde_Aerodinamik_Kuvvetler_N]
  [DCM_s2b] -> Product6/1

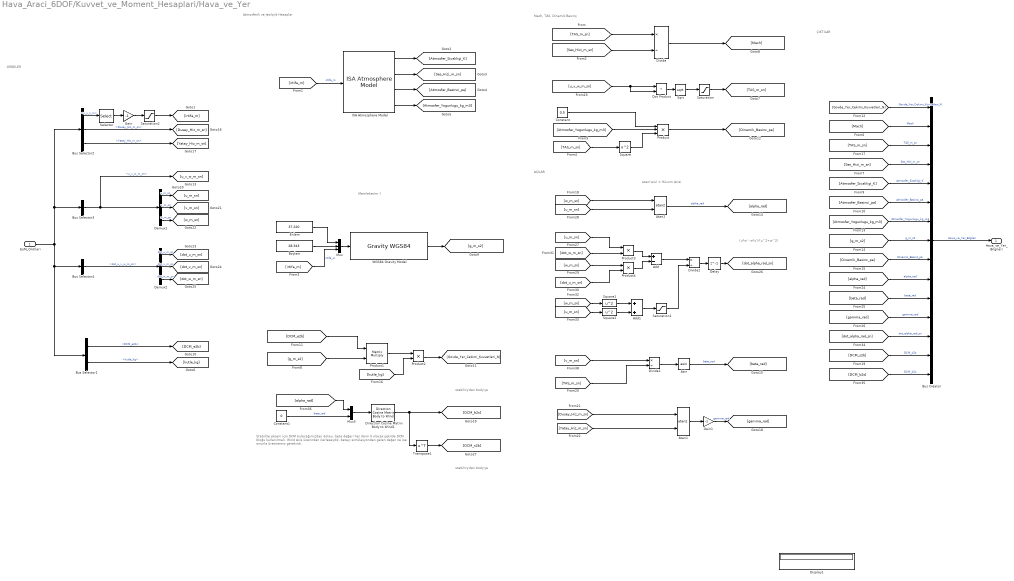
== system Hava_Araci_6DOF/Kuvvet_ve_Moment_Hesaplari/Hava_ve_Yer ==
  note: atan(w/u) = Hücum Acisi
  note: (u*w' - w*u')/(u^2+w^2)
  note: AÇILAR
  note: Memleketim :)
  note: GİRDİLER
  note: ÇIKTILAR
  note: Mach, TAS, Dinamik Basınç
  note: Atmosferik ve Jeolojik Hesaplar
  note: stability'den body'ye
  note: stability'den body'ye
  note: Stabilite ekseni için DCM bulacağımızdan dolayı, bete değeri her daim 0 olacak şekilde DCM bloğu kullanılmalı. Wind Axis üzerinden ilerleseydik, betayı simülasyondan gelen değer ne ise onunla üretmemiz gerekirdi.
  EoM_Ciktilari : Inport  OutDataTypeStr=double
  Add : Sum  Inputs=+-
  Add1 : Sum
  Asin : Trigonometry  Operator=asin
  Atan1 : Trigonometry  Operator=atan2
  Atan2 : Trigonometry  Operator=atan2
  Boylam : Constant  Value=28.343
  Bus Creator : BusCreator  Inputs=15
  Bus Selector1 : BusSelector  OutputSignals=DCM_e2b,kutle_kg
  Bus Selector2 : BusSelector  OutputSignals=x_y_z_m,Dusey_Hiz_m_sn,Yatay_Hiz_m_sn
  Bus Selector3 : BusSelector  OutputSignals=u_v_w_m_sn
  Bus Selector4 : BusSelector  OutputSignals=dot_u_v_w_m_sn
  Constant : Constant  Value=0.5
  Constant1 : Constant  Value=0
  Delay : Delay  DelayLength=1
  Demux1 : Demux  Outputs=3
  Demux2 : Demux  Outputs=3
  Direction Cosine Matrix Body to Wind1 : aerolibtransform2/Direction Cosine Matrix Body to Wind
      settings: SourceProductBaseCode=AE
  Display1 : Display
  Divide : Product  Inputs=*/
  Divide1 : Product  Inputs=*/
  Divide2 : Product  Inputs=*/
  Dot Product : DotProduct  OutDataTypeStr=Inherit: Inherit via internal rule
  Enlem : Constant  Value=37.220
  Gain : Gain  Gain=-1
  Gain1 : Gain  Gain=-1
  ISA Atmosphere Model : aerolibatmos2/ISA Atmosphere Model  custom=off  g=9.80665  gamma=1.4  R=287.0531  L=0.0065  h_trop=11000  h_strat=20000  rho0=1.225  P0=101325  T0=288.15  h0=0
  Mux : Mux  Inputs=3
  Mux3 : Mux  Inputs=2
  Product : Product  Inputs=3
  Product1 : Product  Multiplication=Matrix(*)
  Product2 : Product
  Product3 : Product
  Product4 : Product
  Saturation : Saturate  UpperLimit=inf  LowerLimit=0.000000001
  Saturation1 : Saturate  UpperLimit=inf  LowerLimit=0.000000001
  Saturation2 : Saturate  UpperLimit=inf  LowerLimit=1
  Selector : Selector  InputPortWidth=3  IndexOptions=Index vector (dialog)  Indices=3  OutputSizes=1
  Sqrt : Sqrt
  Square : Math  Operator=square
  Square1 : Math  Operator=square
  Square2 : Math  Operator=square
  Transpose1 : Math  Operator=transpose
  "WGS84 Gravity Model  " : GravityWGS84
  Hava_ve_Yer_Bilgileri : Outport
  wires:
  Bus Creator/1 -> Hava_ve_Yer_Bilgileri/1  "Hava_ve_Yer_Bilgileri"
  EoM_Ciktilari/1 -> Bus Selector1/1, Bus Selector4/1, Bus Selector2/1, Bus Selector3/1
  [irtifa_m] -> ISA Atmosphere Model/1  "irtifa_m"
  Bus Selector2/1 -> Selector/1  "<x_y_z_m>"
  Selector/1 -> Gain/1
  Gain/1 -> Saturation2/1
  ISA Atmosphere Model/1 -> [Atmosfer_Sicakligi_K]
  ISA Atmosphere Model/2 -> [Ses_Hizi_m_sn]
  ISA Atmosphere Model/3 -> [Atmosfer_Basinci_pa]
  ISA Atmosphere Model/4 -> [Atmosfer_Yogunlugu_kg_m3]
  Bus Selector3/1 -> [u_v_w_m_sn], Demux1/1  "<u_v_w_m_sn>"
  [TAS_m_sn] -> Divide/1
  [Ses_Hizi_m_sn] -> Divide/2
  Divide/1 -> [Mach]
  Mux/1 -> "WGS84 Gravity Model  "/1
  Boylam/1 -> Mux/2
  [irtifa_m] -> Mux/3  "irtifa_m"
  Enlem/1 -> Mux/1
  "WGS84 Gravity Model  "/1 -> [g_m_s2]
  Bus Selector1/1 -> [DCM_e2b]  "<DCM_e2b>"
  [DCM_e2b] -> Product1/1
  Product1/1 -> Product2/1
  [TAS_m_sn] -> Square/1
  Constant/1 -> Product/1
  [Atmosfer_Yogunlugu_kg_m3] -> Product/2
  Square/1 -> Product/3
  Product/1 -> [Dinamik_Basinc_pa]
  [Govde_Yer_Cekimi_Kuvvetleri_N] -> Bus Creator/1  "Govde_Yer_Cekimi_Kuvvetleri_N"
  [Mach] -> Bus Creator/2  "Mach"
  [Ses_Hizi_m_sn] -> Bus Creator/4  "Ses_Hizi_m_sn"
  [Atmosfer_Sicakligi_K] -> Bus Creator/5  "Atmosfer_Sicakligi_K"
  [Atmosfer_Basinci_pa] -> Bus Creator/6  "Atmosfer_Basinci_pa"
  [Atmosfer_Yogunlugu_kg_m3] -> Bus Creator/7  "Atmosfer_Yogunlugu_kg_m3"
  [g_m_s2] -> Bus Creator/8  "g_m_s2"
  [Dinamik_Basinc_pa] -> Bus Creator/9  "Dinamik_Basinc_pa"
  [g_m_s2] -> Product1/2
  Bus Selector1/2 -> [kutle_kg]  "<kutle_kg>"
  [kutle_kg] -> Product2/2
  Product2/1 -> [Govde_Yer_Cekimi_Kuvvetleri_N]
  [TAS_m_sn] -> Bus Creator/3  "TAS_m_sn"
  [u_m_sn] -> Atan2/2
  [w_m_sn] -> Atan2/1
  Atan2/1 -> [alpha_rad]  "alpha_rad"
  [v_m_sn] -> Divide1/1
  [TAS_m_sn] -> Divide1/2
  Divide1/1 -> Asin/1
  Asin/1 -> [beta_rad]  "beta_rad"
  Bus Selector2/2 -> [Dusey_Hiz_m_sn]  "<Dusey_Hiz_m_sn>"
  Bus Selector2/3 -> [Yatay_Hiz_m_sn]  "<Yatay_Hiz_m_sn>"
  [Dusey_Hiz_m_sn] -> Atan1/1
  [Yatay_Hiz_m_sn] -> Atan1/2
  Atan1/1 -> Gain1/1
  Gain1/1 -> [gamma_rad]  "gamma_rad"
  Dot Product/1 -> Sqrt/1
  Sqrt/1 -> Saturation/1
  [u_v_w_m_sn] -> Dot Product/2, Dot Product/1
  [alpha_rad] -> Bus Creator/10  "alpha_rad"
  [beta_rad] -> Bus Creator/11  "beta_rad"
  [gamma_rad] -> Bus Creator/12  "gamma_rad"
  Demux1/1 -> [u_m_sn]  "u_m_sn"
  Demux1/2 -> [v_m_sn]  "v_m_sn"
  Demux1/3 -> [w_m_sn]  "w_m_sn"
  Demux2/3 -> [dot_w_m_sn]  "dot_w_m_sn"
  Demux2/2 -> [dot_v_m_sn]  "dot_v_m_sn"
  Demux2/1 -> [dot_u_m_sn]  "dot_u_m_sn"
  Bus Selector4/1 -> Demux2/1  "<dot_u_v_w_m_sn>"
  [u_m_sn] -> Product3/1
  [dot_w_m_sn] -> Product3/2
  [w_m_sn] -> Product4/1
  [dot_u_m_sn] -> Product4/2
  Product3/1 -> Add/1
  Product4/1 -> Add/2
  Add/1 -> Divide2/1
  [w_m_sn] -> Square1/1
  [u_m_sn] -> Square2/1
  Square1/1 -> Add1/1
  Square2/1 -> Add1/2
  Add1/1 -> Saturation1/1
  Divide2/1 -> Delay/1
  [dot_alpha_rad_sn] -> Bus Creator/13  "dot_alpha_rad_sn"
  [DCM_s2b] -> Bus Creator/14  "DCM_s2b"
  Saturation/1 -> [TAS_m_sn]
  Saturation1/1 -> Divide2/2
  Delay/1 -> [dot_alpha_rad_sn]
  Saturation2/1 -> [irtifa_m]
  [DCM_b2s] -> Bus Creator/15  "DCM_b2s"
  Mux3/1 -> Direction Cosine Matrix Body to Wind1/1
  [alpha_rad] -> Mux3/1
  Direction Cosine Matrix Body to Wind1/1 -> Transpose1/1, [DCM_b2s]
  Constant1/1 -> Mux3/2  "beta_rad"
  Transpose1/1 -> [DCM_s2b]

== system Hava_Araci_6DOF/Kuvvet_ve_Moment_Hesaplari/Itki Hesapları ==
  note: ÇIKTILAR
  note: GİRDİLER
  Servo_Bilgileri : Inport  OutDataTypeStr=double
  1-D Lookup Table : Lookup_n-D  NumberOfTableDimensions=1  BreakpointsForDimension1=servo.thrust.limitler.itki_yuzde_per  Table=itki.limitler_N  ExtrapMethod=Clip  InternalRulePriority=Speed  RndMeth=Simplest
  Bus Creator : BusCreator  Inputs=1
  Bus Selector : BusSelector  OutputSignals=itki_per
  Constant : Constant  Value=0
  Mux : Mux  Inputs=3
  Itki_Bilgileri : Outport
  wires:
  Servo_Bilgileri/1 -> Bus Selector/1
  Bus Selector/1 -> [itki_per]  "<itki_per>"
  [itki_per] -> 1-D Lookup Table/1
  1-D Lookup Table/1 -> [itki_N]
  [itki_N] -> Mux/1
  Constant/1 -> Mux/3, Mux/2
  Mux/1 -> Bus Creator/1  "Govde_Itki_Kuvveti_N"
  Bus Creator/1 -> Itki_Bilgileri/1

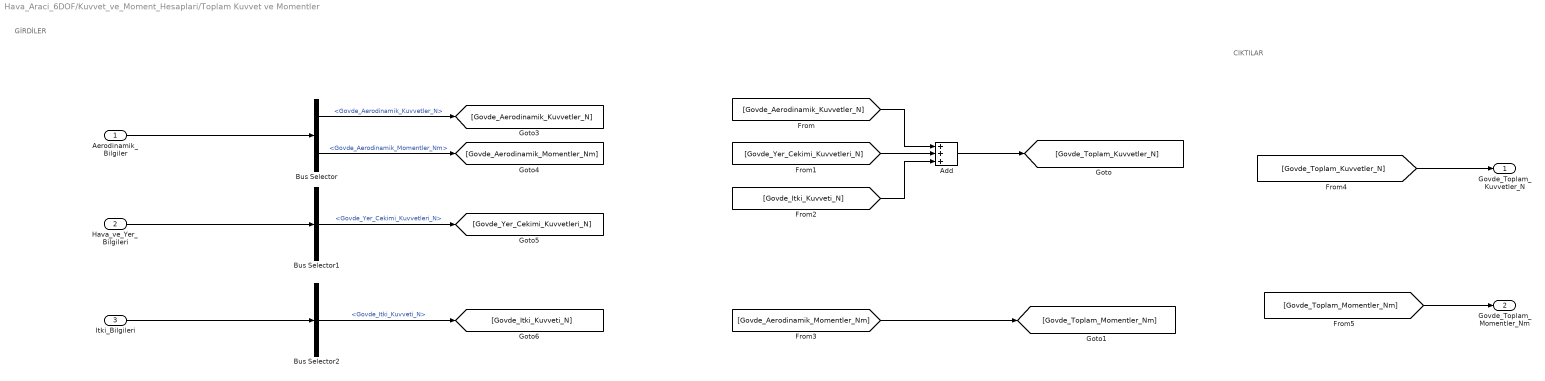
== system Hava_Araci_6DOF/Kuvvet_ve_Moment_Hesaplari/Toplam Kuvvet ve Momentler ==
  note: GİRDİLER
  note: CIKTILAR
  Aerodinamik_Bilgiler : Inport  OutDataTypeStr=double
  Hava_ve_Yer_Bilgileri : Inport  Port=2
  Itki_Bilgileri : Inport  Port=3
  Add : Sum  Inputs=3
  Bus Selector : BusSelector  OutputSignals=Kuvvet_ve_Momentler.Govde_Aerodinamik_Kuvvetler_N,Kuvvet_ve_Momentler.Govde_Aerodinamik_Momentler_Nm
  Bus Selector1 : BusSelector  OutputSignals=Govde_Yer_Cekimi_Kuvvetleri_N
  Bus Selector2 : BusSelector  OutputSignals=Govde_Itki_Kuvveti_N
  Govde_Toplam_Kuvvetler_N : Outport
  Govde_Toplam_Momentler_Nm : Outport  Port=2
  wires:
  Itki_Bilgileri/1 -> Bus Selector2/1
  Hava_ve_Yer_Bilgileri/1 -> Bus Selector1/1
  Aerodinamik_Bilgiler/1 -> Bus Selector/1
  Bus Selector/1 -> [Govde_Aerodinamik_Kuvvetler_N]  "<Govde_Aerodinamik_Kuvvetler_N>"
  Bus Selector/2 -> [Govde_Aerodinamik_Momentler_Nm]  "<Govde_Aerodinamik_Momentler_Nm>"
  Bus Selector1/1 -> [Govde_Yer_Cekimi_Kuvvetleri_N]  "<Govde_Yer_Cekimi_Kuvvetleri_N>"
  Bus Selector2/1 -> [Govde_Itki_Kuvveti_N]  "<Govde_Itki_Kuvveti_N>"
  [Govde_Yer_Cekimi_Kuvvetleri_N] -> Add/2
  [Govde_Aerodinamik_Kuvvetler_N] -> Add/1
  [Govde_Itki_Kuvveti_N] -> Add/3
  Add/1 -> [Govde_Toplam_Kuvvetler_N]
  [Govde_Aerodinamik_Momentler_Nm] -> [Govde_Toplam_Momentler_Nm]
  [Govde_Toplam_Kuvvetler_N] -> Govde_Toplam_Kuvvetler_N/1
  [Govde_Toplam_Momentler_Nm] -> Govde_Toplam_Momentler_Nm/1

== system Hava_Araci_6DOF/Hareket Denklemleri (Equations of Motion)/Acisal_Ivme_Hesaplari/Subsystem ==
  p q r : Inport
  Inertia : Inport  Port=2
  Product : Product  Multiplication=Matrix(*)  InputSameDT=on  SaturateOnIntegerOverflow=on  OutDataTypeStr=Inherit: Same as first input
  Reshape1 : Reshape  OutputDimensionality=Column vector (2-D)
  Reshape2 : Reshape
  I * w : Outport  VectorParamsAs1DForOutWhenUnconnected=off
  wires:
  Product/1 -> Reshape2/1
  Reshape1/1 -> Product/2
  Reshape2/1 -> I * w/1
  p q r/1 -> Reshape1/1
  Inertia/1 -> Product/1

== system Hava_Araci_6DOF/Kuvvet_ve_Moment_Hesaplari/Aerodinamik Hesaplar/CD ==
  In Bus Element6 : Inport  PortName=Hava_Bilgileri  Element=Mach
  In Bus Element1 : Inport  PortName=Hava_Bilgileri  Element=alpha_rad
  Abs : Abs  SaturateOnIntegerOverflow=off
  Add : Sum  Inputs=3
  CD_0 : Lookup_n-D  NumberOfTableDimensions=1  BreakpointsForDimension1=aerodatabase.bps.Mach  Table=aerodatabase.tablolar.CD  ExtrapMethod=Clip  InternalRulePriority=Speed  RndMeth=Simplest
  CD_M : Lookup_n-D  NumberOfTableDimensions=1  BreakpointsForDimension1=aerodatabase.bps.Mach  Table=aerodatabase.tablolar.CD_M  ExtrapMethod=Clip  InternalRulePriority=Speed  RndMeth=Simplest
  CD_a : Lookup_n-D  NumberOfTableDimensions=1  BreakpointsForDimension1=aerodatabase.bps.Mach  Table=aerodatabase.tablolar.CD_a  ExtrapMethod=Clip  InternalRulePriority=Speed  RndMeth=Simplest
  Product : Product
  Product1 : Product
  CD : Outport
  wires:
  CD_a/1 -> Product1/1
  CD_M/1 -> Product/1
  In Bus Element6/1 -> CD_M/1, Product/2, CD_0/1, CD_a/1
  In Bus Element1/1 -> Abs/1
  Product1/1 -> Add/2
  Product/1 -> Add/3
  CD_0/1 -> Add/1
  Add/1 -> CD/1
  Abs/1 -> Product1/2

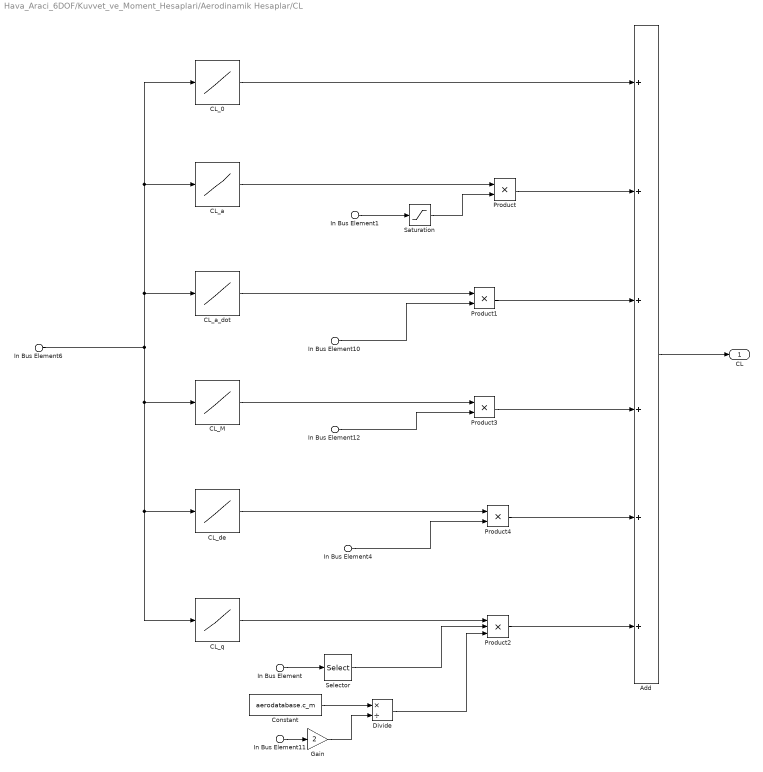
== system Hava_Araci_6DOF/Kuvvet_ve_Moment_Hesaplari/Aerodinamik Hesaplar/CL ==
  In Bus Element : Inport  PortName=EoM_Ciktilari  Element=p_q_r_rad_sn
  In Bus Element1 : Inport  Port=2  PortName=Hava_Bilgileri  Element=alpha_rad
  In Bus Element6 : Inport  Port=2  PortName=Hava_Bilgileri  Element=Mach
  In Bus Element12 : Inport  Port=2  PortName=Hava_Bilgileri  Element=Mach
  In Bus Element10 : Inport  Port=2  PortName=Hava_Bilgileri  Element=dot_alpha_rad_sn
  In Bus Element11 : Inport  Port=2  PortName=Hava_Bilgileri  Element=TAS_m_sn
  In Bus Element4 : Inport  Port=3  PortName=Servo_Bilgileri  Element=elevator_rad
  Add : Sum  Inputs=6
  CL_0 : Lookup_n-D  NumberOfTableDimensions=1  BreakpointsForDimension1=aerodatabase.bps.Mach  Table=aerodatabase.tablolar.CL  ExtrapMethod=Clip  InternalRulePriority=Speed  RndMeth=Simplest
  CL_M : Lookup_n-D  NumberOfTableDimensions=1  BreakpointsForDimension1=aerodatabase.bps.Mach  Table=aerodatabase.tablolar.CL_M  ExtrapMethod=Clip  InternalRulePriority=Speed  RndMeth=Simplest
  CL_a : Lookup_n-D  NumberOfTableDimensions=1  BreakpointsForDimension1=aerodatabase.bps.Mach  Table=aerodatabase.tablolar.CL_a  ExtrapMethod=Clip  InternalRulePriority=Speed  RndMeth=Simplest
  CL_a_dot : Lookup_n-D  NumberOfTableDimensions=1  BreakpointsForDimension1=aerodatabase.bps.Mach  Table=aerodatabase.tablolar.CL_a_dot  ExtrapMethod=Clip  InternalRulePriority=Speed  RndMeth=Simplest
  CL_de : Lookup_n-D  NumberOfTableDimensions=1  BreakpointsForDimension1=aerodatabase.bps.Mach  Table=aerodatabase.tablolar.CL_de  ExtrapMethod=Clip  InternalRulePriority=Speed  RndMeth=Simplest
  CL_q : Lookup_n-D  NumberOfTableDimensions=1  BreakpointsForDimension1=aerodatabase.bps.Mach  Table=aerodatabase.tablolar.CL_q  ExtrapMethod=Clip  InternalRulePriority=Speed  RndMeth=Simplest
  Constant : Constant  Value=aerodatabase.c_m
  Divide : Product  Inputs=*/
  Gain : Gain  Gain=2
  Product{,1,3..4} (4 alike) : Product
  Product2 : Product  Inputs=3
  Saturation : Saturate  UpperLimit=aerodatabase.limitler.alpha_rad(2)  LowerLimit=aerodatabase.limitler.alpha_rad(1)
  Selector : Selector  InputPortWidth=3  IndexOptions=Index vector (dialog)  Indices=[2]  OutputSizes=1
  CL : Outport
  wires:
  CL_0/1 -> Add/1
  CL_de/1 -> Product4/1
  CL_M/1 -> Product3/1
  CL_a/1 -> Product/1
  CL_a_dot/1 -> Product1/1
  In Bus Element1/1 -> Saturation/1
  Saturation/1 -> Product/2
  In Bus Element10/1 -> Product1/2
  In Bus Element/1 -> Selector/1
  Selector/1 -> Product2/2
  CL_q/1 -> Product2/1
  Constant/1 -> Divide/1
  In Bus Element11/1 -> Gain/1
  Gain/1 -> Divide/2
  Divide/1 -> Product2/3
  In Bus Element12/1 -> Product3/2
  In Bus Element4/1 -> Product4/2
  Product/1 -> Add/2
  Product1/1 -> Add/3
  Product4/1 -> Add/5
  Product3/1 -> Add/4
  Product2/1 -> Add/6
  In Bus Element6/1 -> CL_q/1, CL_de/1, CL_M/1, CL_0/1, CL_a/1, CL_a_dot/1
  Add/1 -> CL/1

== system Hava_Araci_6DOF/Kuvvet_ve_Moment_Hesaplari/Aerodinamik Hesaplar/CY ==
  In Bus Element12 : Inport  PortName=Hava_Bilgileri  Element=Mach
  In Bus Element : Inport  PortName=Hava_Bilgileri  Element=beta_rad
  In Bus Element1 : Inport  Port=2  PortName=Servo_Bilgileri  Element=rudder_rad
  Add : Sum
  Cy_B : Lookup_n-D  NumberOfTableDimensions=1  BreakpointsForDimension1=aerodatabase.bps.Mach  Table=aerodatabase.tablolar.Cy_B  ExtrapMethod=Clip  InternalRulePriority=Speed  RndMeth=Simplest
  Cy_dr : Lookup_n-D  NumberOfTableDimensions=1  BreakpointsForDimension1=aerodatabase.bps.Mach  Table=aerodatabase.tablolar.Cy_dr  ExtrapMethod=Clip  InternalRulePriority=Speed  RndMeth=Simplest
  Product : Product
  Product1 : Product
  CY : Outport
  wires:
  Cy_dr/1 -> Product/1
  In Bus Element12/1 -> Cy_dr/1, Cy_B/1
  In Bus Element1/1 -> Product/2
  In Bus Element/1 -> Product1/2
  Product1/1 -> Add/1
  Product/1 -> Add/2
  Add/1 -> CY/1
  Cy_B/1 -> Product1/1

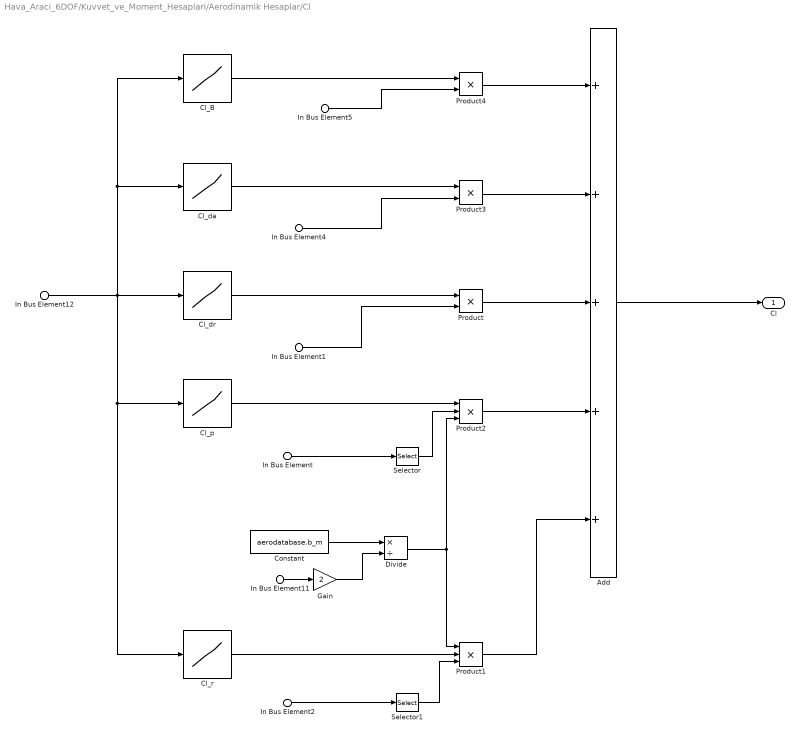
== system Hava_Araci_6DOF/Kuvvet_ve_Moment_Hesaplari/Aerodinamik Hesaplar/Cl ==
  In Bus Element : Inport  PortName=EoM_Ciktilari  Element=p_q_r_rad_sn
  In Bus Element2 : Inport  PortName=EoM_Ciktilari  Element=p_q_r_rad_sn
  In Bus Element12 : Inport  Port=2  PortName=Hava_Bilgileri  Element=Mach
  In Bus Element11 : Inport  Port=2  PortName=Hava_Bilgileri  Element=TAS_m_sn
  In Bus Element5 : Inport  Port=2  PortName=Hava_Bilgileri  Element=beta_rad
  In Bus Element1 : Inport  Port=3  PortName=Servo_Bilgileri  Element=rudder_rad
  In Bus Element4 : Inport  Port=3  PortName=Servo_Bilgileri  Element=aileron_rad
  Add : Sum  Inputs=5
  Cl_B : Lookup_n-D  NumberOfTableDimensions=1  BreakpointsForDimension1=aerodatabase.bps.Mach  Table=aerodatabase.tablolar.Cl_B  ExtrapMethod=Clip  InternalRulePriority=Speed  RndMeth=Simplest
  Cl_da : Lookup_n-D  NumberOfTableDimensions=1  BreakpointsForDimension1=aerodatabase.bps.Mach  Table=aerodatabase.tablolar.Cl_da  ExtrapMethod=Clip  InternalRulePriority=Speed  RndMeth=Simplest
  Cl_dr : Lookup_n-D  NumberOfTableDimensions=1  BreakpointsForDimension1=aerodatabase.bps.Mach  Table=aerodatabase.tablolar.Cl_dr  ExtrapMethod=Clip  InternalRulePriority=Speed  RndMeth=Simplest
  Cl_p : Lookup_n-D  NumberOfTableDimensions=1  BreakpointsForDimension1=aerodatabase.bps.Mach  Table=aerodatabase.tablolar.Cl_p  ExtrapMethod=Clip  InternalRulePriority=Speed  RndMeth=Simplest
  Cl_r : Lookup_n-D  NumberOfTableDimensions=1  BreakpointsForDimension1=aerodatabase.bps.Mach  Table=aerodatabase.tablolar.Cl_r  ExtrapMethod=Clip  InternalRulePriority=Speed  RndMeth=Simplest
  Constant : Constant  Value=aerodatabase.b_m
  Divide : Product  Inputs=*/
  Gain : Gain  Gain=2
  Product : Product
  Product1 : Product  Inputs=3
  Product2 : Product  Inputs=3
  Product3 : Product
  Product4 : Product
  Selector : Selector  InputPortWidth=3  IndexOptions=Index vector (dialog)  Indices=1  OutputSizes=1
  Selector1 : Selector  InputPortWidth=3  IndexOptions=Index vector (dialog)  Indices=3  OutputSizes=1
  Cl : Outport
  wires:
  Cl_da/1 -> Product3/1
  Cl_p/1 -> Product2/1
  Cl_B/1 -> Product4/1
  In Bus Element12/1 -> Cl_B/1, Cl_da/1, Cl_r/1, Cl_p/1, Cl_dr/1
  Cl_dr/1 -> Product/1
  In Bus Element/1 -> Selector/1
  In Bus Element1/1 -> Product/2
  Selector/1 -> Product2/2
  Constant/1 -> Divide/1
  In Bus Element11/1 -> Gain/1
  Gain/1 -> Divide/2
  Divide/1 -> Product2/3, Product1/1
  In Bus Element2/1 -> Selector1/1
  Cl_r/1 -> Product1/2
  Selector1/1 -> Product1/3
  In Bus Element4/1 -> Product3/2
  In Bus Element5/1 -> Product4/2
  Product4/1 -> Add/1
  Product3/1 -> Add/2
  Product/1 -> Add/3
  Product2/1 -> Add/4
  Product1/1 -> Add/5
  Add/1 -> Cl/1

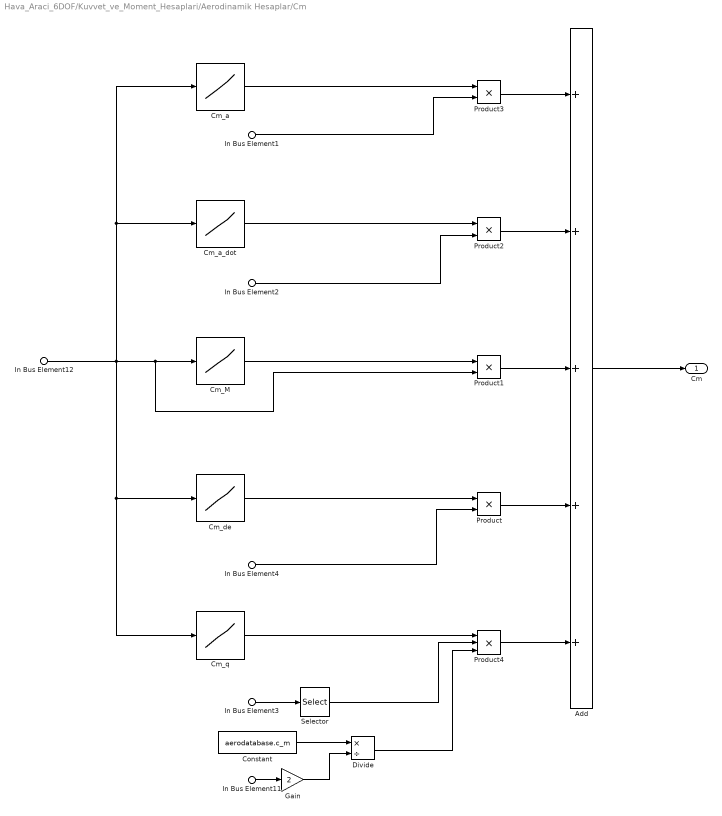
== system Hava_Araci_6DOF/Kuvvet_ve_Moment_Hesaplari/Aerodinamik Hesaplar/Cm ==
  In Bus Element3 : Inport  PortName=EoM_Ciktilari  Element=p_q_r_rad_sn
  In Bus Element12 : Inport  Port=2  PortName=Hava_Bilgileri  Element=Mach
  In Bus Element1 : Inport  Port=2  PortName=Hava_Bilgileri  Element=alpha_rad
  In Bus Element2 : Inport  Port=2  PortName=Hava_Bilgileri  Element=dot_alpha_rad_sn
  In Bus Element11 : Inport  Port=2  PortName=Hava_Bilgileri  Element=TAS_m_sn
  In Bus Element4 : Inport  Port=3  PortName=Servo_Bilgileri  Element=elevator_rad
  Add : Sum  Inputs=5
  Cm_M : Lookup_n-D  NumberOfTableDimensions=1  BreakpointsForDimension1=aerodatabase.bps.Mach  Table=aerodatabase.tablolar.Cm_M  ExtrapMethod=Clip  InternalRulePriority=Speed  RndMeth=Simplest
  Cm_a : Lookup_n-D  NumberOfTableDimensions=1  BreakpointsForDimension1=aerodatabase.bps.Mach  Table=aerodatabase.tablolar.Cm_a  ExtrapMethod=Clip  InternalRulePriority=Speed  RndMeth=Simplest
  Cm_a_dot : Lookup_n-D  NumberOfTableDimensions=1  BreakpointsForDimension1=aerodatabase.bps.Mach  Table=aerodatabase.tablolar.Cm_a_dot  ExtrapMethod=Clip  InternalRulePriority=Speed  RndMeth=Simplest
  Cm_de : Lookup_n-D  NumberOfTableDimensions=1  BreakpointsForDimension1=aerodatabase.bps.Mach  Table=aerodatabase.tablolar.Cm_de  ExtrapMethod=Clip  InternalRulePriority=Speed  RndMeth=Simplest
  Cm_q : Lookup_n-D  NumberOfTableDimensions=1  BreakpointsForDimension1=aerodatabase.bps.Mach  Table=aerodatabase.tablolar.Cm_q  ExtrapMethod=Clip  InternalRulePriority=Speed  RndMeth=Simplest
  Constant : Constant  Value=aerodatabase.c_m
  Divide : Product  Inputs=*/
  Gain : Gain  Gain=2
  Product{,1..3} (4 alike) : Product
  Product4 : Product  Inputs=3
  Selector : Selector  InputPortWidth=3  IndexOptions=Index vector (dialog)  Indices=[2]  OutputSizes=1
  Cm : Outport
  wires:
  In Bus Element12/1 -> Cm_q/1, Cm_de/1, Product1/2, Cm_M/1, Cm_a/1, Cm_a_dot/1
  Cm_de/1 -> Product/1
  In Bus Element4/1 -> Product/2
  Cm_M/1 -> Product1/1
  Cm_a_dot/1 -> Product2/1
  In Bus Element2/1 -> Product2/2
  Cm_a/1 -> Product3/1
  In Bus Element1/1 -> Product3/2
  Constant/1 -> Divide/1
  Selector/1 -> Product4/2
  In Bus Element3/1 -> Selector/1
  In Bus Element11/1 -> Gain/1
  Divide/1 -> Product4/3
  Gain/1 -> Divide/2
  Cm_q/1 -> Product4/1
  Product3/1 -> Add/1
  Product2/1 -> Add/2
  Product1/1 -> Add/3
  Product/1 -> Add/4
  Product4/1 -> Add/5
  Add/1 -> Cm/1

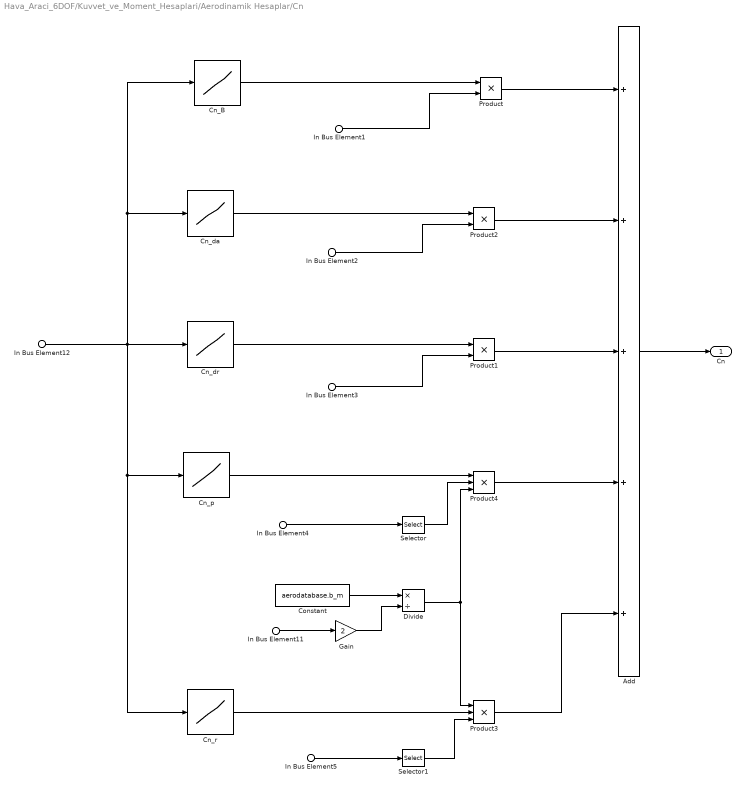
== system Hava_Araci_6DOF/Kuvvet_ve_Moment_Hesaplari/Aerodinamik Hesaplar/Cn ==
  In Bus Element4 : Inport  PortName=EoM_Ciktilari  Element=p_q_r_rad_sn
  In Bus Element5 : Inport  PortName=EoM_Ciktilari  Element=p_q_r_rad_sn
  In Bus Element12 : Inport  Port=2  PortName=Hava_Bilgileri  Element=Mach
  In Bus Element1 : Inport  Port=2  PortName=Hava_Bilgileri  Element=beta_rad
  In Bus Element11 : Inport  Port=2  PortName=Hava_Bilgileri  Element=TAS_m_sn
  In Bus Element2 : Inport  Port=3  PortName=Servo_Bilgileri  Element=aileron_rad
  In Bus Element3 : Inport  Port=3  PortName=Servo_Bilgileri  Element=rudder_rad
  Add : Sum  Inputs=5
  Cn_B : Lookup_n-D  NumberOfTableDimensions=1  BreakpointsForDimension1=aerodatabase.bps.Mach  Table=aerodatabase.tablolar.Cn_B  ExtrapMethod=Clip  InternalRulePriority=Speed  RndMeth=Simplest
  Cn_da : Lookup_n-D  NumberOfTableDimensions=1  BreakpointsForDimension1=aerodatabase.bps.Mach  Table=aerodatabase.tablolar.Cn_da  ExtrapMethod=Clip  InternalRulePriority=Speed  RndMeth=Simplest
  Cn_dr : Lookup_n-D  NumberOfTableDimensions=1  BreakpointsForDimension1=aerodatabase.bps.Mach  Table=aerodatabase.tablolar.Cn_dr  ExtrapMethod=Clip  InternalRulePriority=Speed  RndMeth=Simplest
  Cn_p : Lookup_n-D  NumberOfTableDimensions=1  BreakpointsForDimension1=aerodatabase.bps.Mach  Table=aerodatabase.tablolar.Cn_p  ExtrapMethod=Clip  InternalRulePriority=Speed  RndMeth=Simplest
  Cn_r : Lookup_n-D  NumberOfTableDimensions=1  BreakpointsForDimension1=aerodatabase.bps.Mach  Table=aerodatabase.tablolar.Cn_r  ExtrapMethod=Clip  InternalRulePriority=Speed  RndMeth=Simplest
  Constant : Constant  Value=aerodatabase.b_m
  Divide : Product  Inputs=*/
  Gain : Gain  Gain=2
  Product : Product
  Product1 : Product
  Product2 : Product
  Product3 : Product  Inputs=3
  Product4 : Product  Inputs=3
  Selector : Selector  InputPortWidth=3  IndexOptions=Index vector (dialog)  Indices=1  OutputSizes=1
  Selector1 : Selector  InputPortWidth=3  IndexOptions=Index vector (dialog)  Indices=3  OutputSizes=1
  Cn : Outport
  wires:
  Cn_B/1 -> Product/1
  In Bus Element1/1 -> Product/2
  Cn_dr/1 -> Product1/1
  In Bus Element3/1 -> Product1/2
  Cn_da/1 -> Product2/1
  In Bus Element2/1 -> Product2/2
  In Bus Element12/1 -> Cn_da/1, Cn_B/1, Cn_r/1, Cn_p/1, Cn_dr/1
  Selector1/1 -> Product3/3
  Divide/1 -> Product3/1, Product4/3
  Cn_r/1 -> Product3/2
  Selector/1 -> Product4/2
  Constant/1 -> Divide/1
  In Bus Element4/1 -> Selector/1
  Cn_p/1 -> Product4/1
  In Bus Element11/1 -> Gain/1
  In Bus Element5/1 -> Selector1/1
  Gain/1 -> Divide/2
  Product3/1 -> Add/5
  Product2/1 -> Add/2
  Product4/1 -> Add/4
  Product1/1 -> Add/3
  Product/1 -> Add/1
  Add/1 -> Cn/1
